simulink model "MR2_AndoidIPApplication"  (R2018b)
settings: Solver=VariableStepAuto  StartTime=0.0  StopTime=10.0  RelTol=1e-3
undefined symbols (not defined in the file): Backcamfinal, BLE_Send, LightIntensity, Line_Detection, LineDirection, Rec, SandDune, SDTV
libraries: androiduilib x8, androidaudiovideolib x2, visiontransforms x2, androidcommunicationlib x1, visionconversions x1, visionanalysis x1, visionstatistics x1, androidsensorlib x1, visiontextngfix x1
settings Model: Creator=Darshan  LastModifiedBy=Darshan

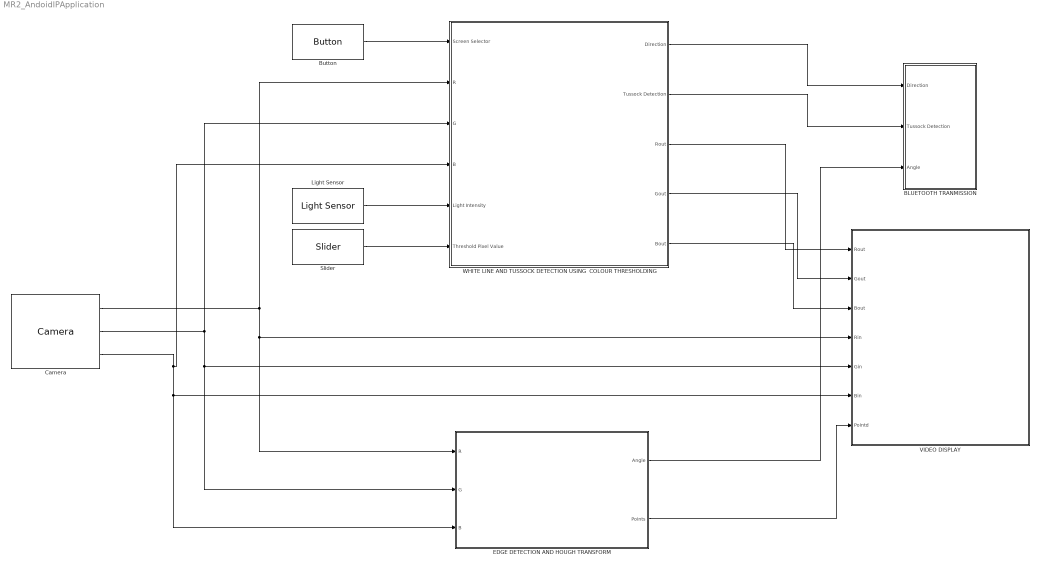
== system MR2_AndoidIPApplication ==
  BLUETOOTH TRANMISSION : Subsystem
  Button : androiduilib/Button  ButtonState=Not pressed  ButtonId=Backcamfinal/Button  State=off  SampleTime=0.1  BlockPlatform=Android
      settings: SourceProductName=Simulink Support Package for Android Devices  SourceProductBaseCode=ANDROID
  Camera : androidaudiovideolib/Camera  CameraLocation=Back  CameraResolutions=Back - 640x480  Width=640  Height=480  SampleTime=0.1  BlockPlatform=Android
      settings: SourceProductName=Simulink Support Package for Android Devices  SourceProductBaseCode=ANDROID
  "EDGE DETECTION AND HOUGH TRANSFORM " : Subsystem
  Light Sensor : androidsensorlib/Light Sensor  SampleTime=0.1  BlockPlatform=Android
      settings: SourceProductName=Simulink Support Package for Android Devices  SourceProductBaseCode=ANDROID
  Slider : androiduilib/Slider  Min=10000  Value=75000  Max=150000  Resolution=1  SliderId=Backcamfinal/Slider  SampleTime=0.1  BlockPlatform=Android
      settings: SourceProductName=Simulink Support Package for Android Devices  SourceProductBaseCode=ANDROID
  VIDEO DISPLAY : Subsystem
  WHITE LINE AND TUSSOCK DETECTION USING  COLOUR THRESHOLDING : Subsystem
  wires:
  "EDGE DETECTION AND HOUGH TRANSFORM "/2(Points) -> VIDEO DISPLAY/7(Pointd)
  WHITE LINE AND TUSSOCK DETECTION USING  COLOUR THRESHOLDING/5(Bout) -> VIDEO DISPLAY/3(Bout)
  WHITE LINE AND TUSSOCK DETECTION USING  COLOUR THRESHOLDING/3(Rout) -> VIDEO DISPLAY/1(Rout)
  WHITE LINE AND TUSSOCK DETECTION USING  COLOUR THRESHOLDING/2(Tussock Detection) -> BLUETOOTH TRANMISSION/2(Tussock Detection)
  WHITE LINE AND TUSSOCK DETECTION USING  COLOUR THRESHOLDING/1(Direction) -> BLUETOOTH TRANMISSION/1(Direction)
  Camera/3 -> "EDGE DETECTION AND HOUGH TRANSFORM "/3(B), VIDEO DISPLAY/6(Bin), WHITE LINE AND TUSSOCK DETECTION USING  COLOUR THRESHOLDING/4(B)
  Light Sensor/1 -> WHITE LINE AND TUSSOCK DETECTION USING  COLOUR THRESHOLDING/5(Light Intensity)
  Button/1 -> WHITE LINE AND TUSSOCK DETECTION USING  COLOUR THRESHOLDING/1(Screen Selector)
  Slider/1 -> WHITE LINE AND TUSSOCK DETECTION USING  COLOUR THRESHOLDING/6(Threshold Pixel Value)
  Camera/2 -> "EDGE DETECTION AND HOUGH TRANSFORM "/2(G), VIDEO DISPLAY/5(Gin), WHITE LINE AND TUSSOCK DETECTION USING  COLOUR THRESHOLDING/3(G)
  Camera/1 -> "EDGE DETECTION AND HOUGH TRANSFORM "/1(R), VIDEO DISPLAY/4(Rin), WHITE LINE AND TUSSOCK DETECTION USING  COLOUR THRESHOLDING/2(R)
  "EDGE DETECTION AND HOUGH TRANSFORM "/1("Angle ") -> BLUETOOTH TRANMISSION/3("Angle ")
  WHITE LINE AND TUSSOCK DETECTION USING  COLOUR THRESHOLDING/4(Gout) -> VIDEO DISPLAY/2(Gout)

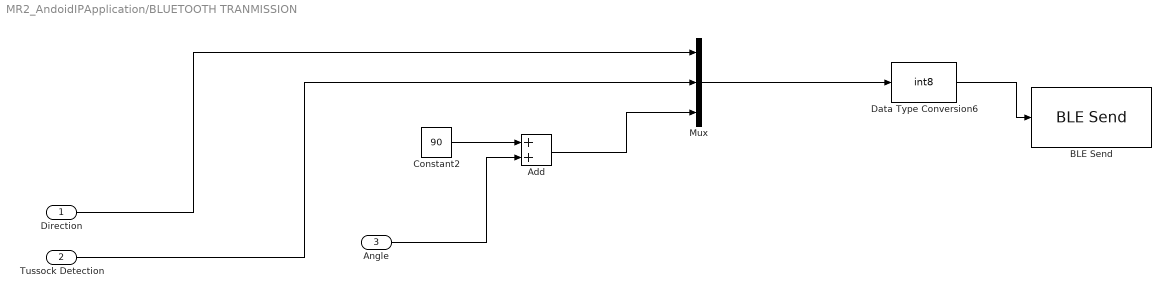
== system MR2_AndoidIPApplication/BLUETOOTH TRANMISSION ==
  Direction : Inport
  Tussock Detection : Inport  Port=2
  "Angle " : Inport  Port=3
  Add : Sum
  BLE Send : androidcommunicationlib/BLE Send  DeviceMode=Central (Client)  BluetoothAddress=00:15:85:14:9C:09  CharUUID=0000ffe1-0000-1000-8000-00805f9b34fb  ServiceUUID=0000ffe0-0000-1000-8000-00805f9b34fb  device=BT05  character=0000ffe0-0000-1000-8000-00805f9b34fb\0000ffe1-0000-1000-8000-00805f9b34fb  CustomService=off  ServiceName=Heart Rate  CharacteristicName="Heart Rate  Measurement"  CustomServiceUUID=<Enter Service UUID>  CustomCharUUID=<Enter Characteristic UUID>  charseruuid=00001800-0000-1000-8000-00805f9b34fb\00002a00-0000-1000-8000-00805f9b34fb  seruuid=00001810-0000-1000-8000-00805f9b34fb  chruuid=00002a37-0000-1000-8000-00805f9b34fb  PeripheralService=0000180d-0000-1000-8000-00805f9b34fb  PeripheralCharacteristic=00002a37-0000-1000-8000-00805f9b34fb  BLEId=Backcamfinal/BLE_Send  Devicename=BT05  IsCustomService=0  Size=-1
      settings: SourceProductName=Simulink Support Package for Android Devices  SourceProductBaseCode=ANDROID
  Constant2 : Constant  Value=90
  Data Type Conversion6 : DataTypeConversion  OutDataTypeStr=int8
  Mux : Mux  Inputs=3
  wires:
  Tussock Detection/1 -> Mux/2
  Constant2/1 -> Add/1
  Add/1 -> Mux/3
  Data Type Conversion6/1 -> BLE Send/1
  Direction/1 -> Mux/1
  Mux/1 -> Data Type Conversion6/1
  "Angle "/1 -> Add/2

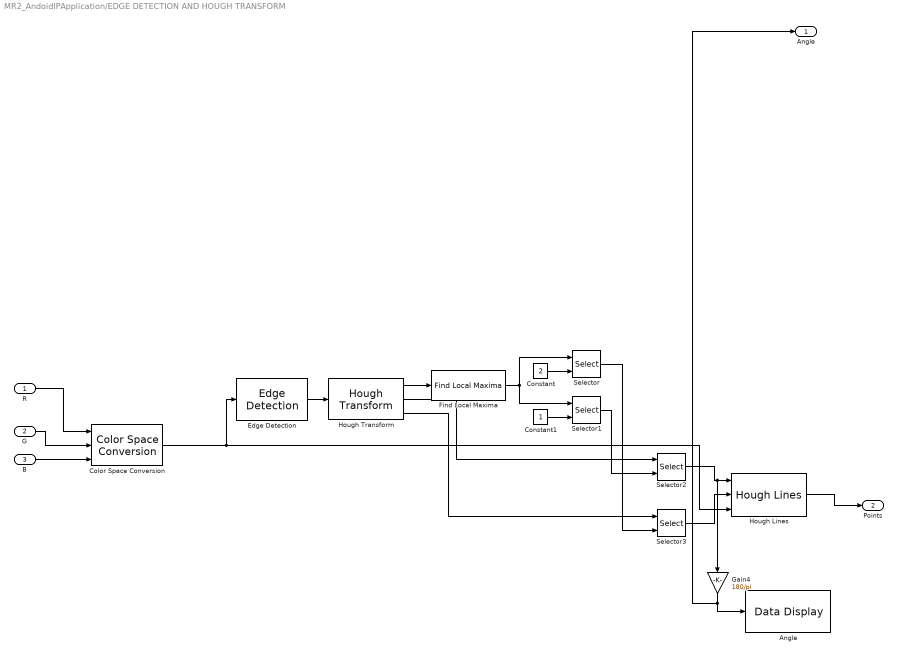
== system MR2_AndoidIPApplication/EDGE DETECTION AND HOUGH TRANSFORM  ==
  R : Inport
  G : Inport  Port=2
  B : Inport  Port=3
  Angle : androiduilib/Data Display  DataDisplayId=Backcamfinal/Angle  Format=Float  Precision=6  SimulateUsing=Code generation  blockPlatform=Android
      settings: SourceProductName=Simulink Support Package for Android Devices  SourceProductBaseCode=ANDROID
  Color Space Conversion : visionconversions/Color Space  Conversion  conversion=Obsolete  conversionActive=R'G'B' to intensity  wp_str=D65  rec=Rec. 601 (SDTV)  sys=1125/60/2:1  imagePorts=Separate color signals
      settings: SourceProductName=Computer Vision System Toolbox
  Constant : Constant  Value=2
  Constant1 : Constant
  Edge Detection : visionanalysis/Edge Detection  method=Sobel  outputType=Binary image  userDefinedThreshold=off  thresholdSource=Input port  threshold=20  thresholdTuning=10  edgeThinning=off  threshold_canny=[0.25 0.60]  autoPercent=70  sigma=1  roundingMode=Floor  overflowMode=off  prodOutputMode=Binary point scaling  prodOutputWordLength=32  prodOutputFracLength=8  prodOutputSlope=2^-8  accumSlope=2^-8  outputSlope=2^-4
      settings: SourceProductName=Computer Vision System Toolbox  SourceProductBaseCode=VP
  Find Local Maxima : visionstatistics/Find Local Maxima  num_peaks=1  nhood_size=[5 7]  src_thresh=Obsolete9b  src_thresh_inuse=Specify via dialog  threshold=10  inputIsHough=on  dt_peak=uint32  isOutVarDim=on  dt_count=uint32
      settings: SourceProductName=Computer Vision System Toolbox  SourceProductBaseCode=VP
  Gain4 : Gain  Gain=180/pi
  Hough Lines : visiontransforms/Hough Lines  sineCompMethod=Trigonometric function  thetaRes=pi/180  firstCoeffMode=Specify word length  firstCoeffWordLength=16  firstCoeffFracLength=15  prodOutputMode=Binary point scaling  prodOutputWordLength=32  prodOutputFracLength=16  roundingMode=Nearest  overflowMode=on
      settings: SourceProductName=Computer Vision System Toolbox  SourceProductBaseCode=VP
  Hough Transform : visiontransforms/Hough Transform  theta_res=pi/360  rho_res=1  out_theta_rho=on  outdtmode=double  roundingMode=Nearest  overflowMode=on  firstCoeffMode=Binary point scaling  firstCoeffWordLength=16  firstCoeffFracLength=14  firstCoeffSlope=2^-14  secondCoeffMode=Binary point scaling  secondCoeffWordLength=32  secondCoeffFracLength=16  secondCoeffSlope=2^-16  prodOutputMode=Binary point scaling  prodOutputWordLength=32  prodOutputFracLength=20  prodOutputSlope=2^-20  accumMode=Binary point scaling  accumWordLength=32  accumFracLength=20  accumSlope=2^-20  outputMode=Binary point scaling  outputWordLength=16  outputFracLength=0  outputSlope=2^0  memoryMode=Binary point scaling  memoryWordLength=32  memoryFracLength=16  memorySlope=2^-16
      settings: SourceProductName=Computer Vision System Toolbox  SourceProductBaseCode=VP
  Selector : Selector  InputPortWidth=2  IndexOptions=Index vector (port)  Indices=1  OutputSizes=1
  Selector1 : Selector  InputPortWidth=2  IndexOptions=Index vector (port)  Indices=0  OutputSizes=1
  Selector2 : Selector  NumberOfDimensions=2  InputPortWidth=3  IndexOptions=Select all,Index vector (port)  Indices=[1 3],1  OutputSizes=1,1
  Selector3 : Selector  NumberOfDimensions=2  InputPortWidth=3  IndexOptions=Select all,Index vector (port)  Indices=[1 3],1  OutputSizes=1,1
  "Angle " : Outport
  Points : Outport  Port=2
  wires:
  Edge Detection/1 -> Hough Transform/1
  Constant/1 -> Selector/2
  Color Space Conversion/1 -> Hough Lines/3, Edge Detection/1
  Hough Transform/2 -> Selector2/1
  Selector/1 -> Selector3/2
  Selector1/1 -> Selector2/2
  Hough Transform/3 -> Selector3/1
  Constant1/1 -> Selector1/2
  Find Local Maxima/1 -> Selector1/1, Selector/1
  Hough Transform/1 -> Find Local Maxima/1
  Selector2/1 -> Gain4/1, Hough Lines/1
  Gain4/1 -> Angle/1, "Angle "/1
  Selector3/1 -> Hough Lines/2
  R/1 -> Color Space Conversion/1
  G/1 -> Color Space Conversion/2
  B/1 -> Color Space Conversion/3
  Hough Lines/1 -> Points/1

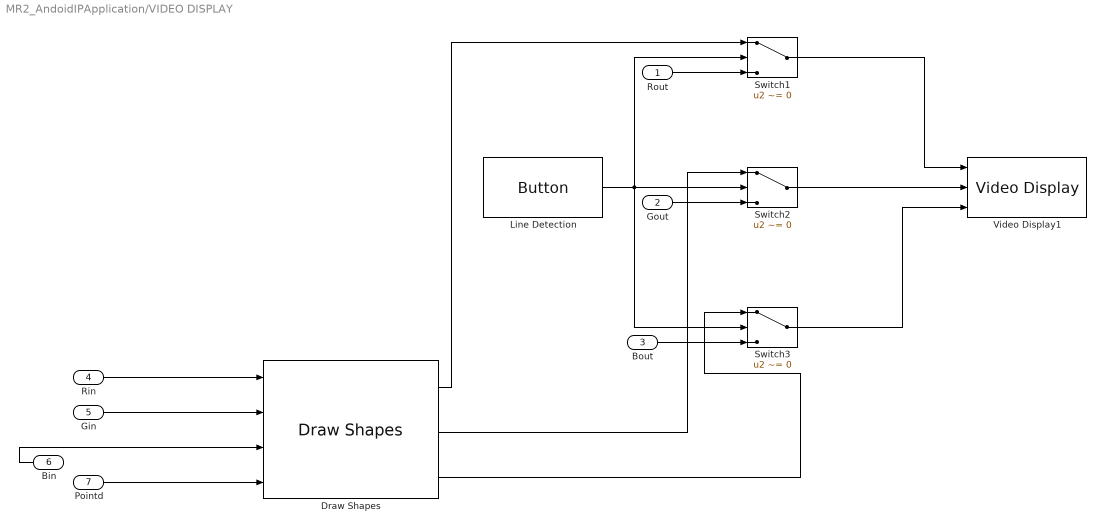
== system MR2_AndoidIPApplication/VIDEO DISPLAY ==
  Rout : Inport
  Gout : Inport  Port=2
  Bout : Inport  Port=3
  Rin : Inport  Port=4
  Gin : Inport  Port=5
  Bin : Inport  Port=6
  Pointd : Inport  Port=7
  Draw Shapes : visiontextngfix/Draw Shapes  shape=Lines  fill=off  lineWidth=5  fillClrSource=Specify via dialog  display=User-specified value  intensity=200  color=[0 255 0]  opacity=0.6  viewport=Entire image  antialiasing=off  inType=Obsolete  imagePorts=Separate color signals  prodOutputMode=Binary point scaling  prodOutputWordLength=32  prodOutputFracLength=14  memoryMode=Specify word length  memoryWordLength=16  memoryFracLength=14  roundingMode=Floor  overflowMode=off
      settings: SourceProductName=Computer Vision System Toolbox
  Line Detection : androiduilib/Button  ButtonState=Not pressed  ButtonId=Backcamfinal/Line_Detection  State=off  SampleTime=0.1  BlockPlatform=Android
      settings: SourceProductName=Simulink Support Package for Android Devices  SourceProductBaseCode=ANDROID
  Switch1 : Switch  Criteria=u2 ~= 0
  Switch2 : Switch  Criteria=u2 ~= 0
  Switch3 : Switch  Criteria=u2 ~= 0
  Video Display1 : androidaudiovideolib/Video Display  BlockPlatform=Android
      settings: SourceProductName=Simulink Support Package for Android Devices  SourceProductBaseCode=ANDROID
  wires:
  Switch1/1 -> Video Display1/1
  Switch3/1 -> Video Display1/3
  Gin/1 -> Draw Shapes/2
  Switch2/1 -> Video Display1/2
  Line Detection/1 -> Switch1/2, Switch2/2, Switch3/2
  Rin/1 -> Draw Shapes/1
  Draw Shapes/2 -> Switch2/1
  Draw Shapes/1 -> Switch1/1
  Draw Shapes/3 -> Switch3/1
  Pointd/1 -> Draw Shapes/4
  Rout/1 -> Switch1/3
  Bout/1 -> Switch3/3
  Gout/1 -> Switch2/3
  Bin/1 -> Draw Shapes/3

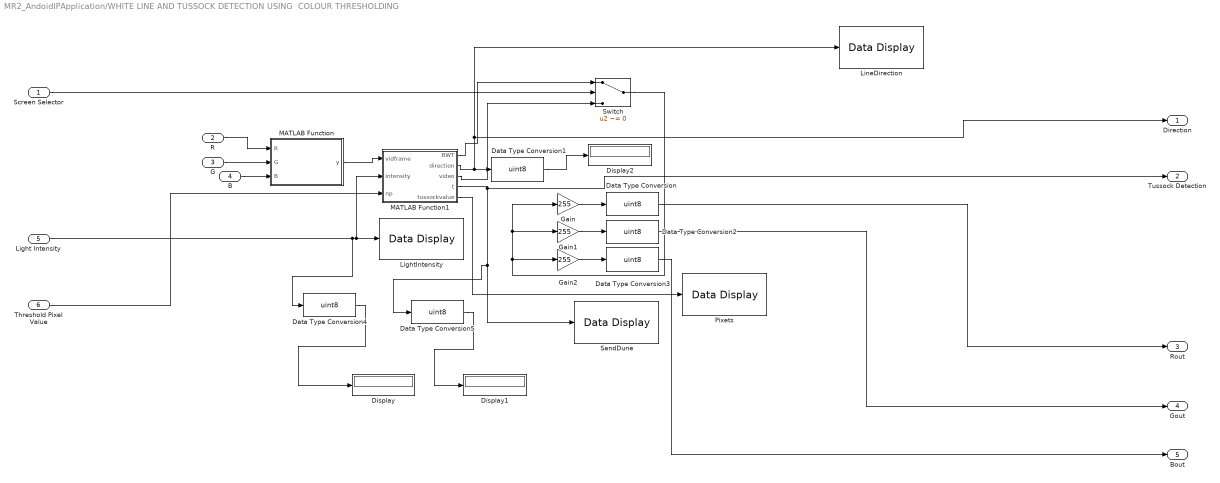
== system MR2_AndoidIPApplication/WHITE LINE AND TUSSOCK DETECTION USING  COLOUR THRESHOLDING ==
  Screen Selector : Inport
  R : Inport  Port=2
  G : Inport  Port=3
  B : Inport  Port=4
  Light Intensity : Inport  Port=5
  Threshold Pixel Value : Inport  Port=6
  Data Type Conversion{,1..5} (6 alike) : DataTypeConversion  OutDataTypeStr=uint8
  Display : Display
  Display1 : Display
  Display2 : Display
  Gain : Gain  Gain=255
  Gain1 : Gain  Gain=255
  Gain2 : Gain  Gain=255
  LightIntensity : androiduilib/Data Display  DataDisplayId=Backcamfinal/LightIntensity  Format=Float  Precision=6  SimulateUsing=Code generation  blockPlatform=Android
      settings: SourceProductName=Simulink Support Package for Android Devices  SourceProductBaseCode=ANDROID
  LineDirection : androiduilib/Data Display  DataDisplayId=Backcamfinal/LineDirection  Format=Float  Precision=6  SimulateUsing=Code generation  blockPlatform=Android
      settings: SourceProductName=Simulink Support Package for Android Devices  SourceProductBaseCode=ANDROID
  MATLAB Function : MATLAB Function  TreatAsAtomicUnit=on
  MATLAB Function1 : MATLAB Function  TreatAsAtomicUnit=on
  Pixets : androiduilib/Data Display  DataDisplayId=Backcamfinal/Pixets  Format=Float  Precision=6  SimulateUsing=Code generation  blockPlatform=Android
      settings: SourceProductName=Simulink Support Package for Android Devices  SourceProductBaseCode=ANDROID
  SandDune : androiduilib/Data Display  DataDisplayId=Backcamfinal/SandDune  Format=Float  Precision=6  SimulateUsing=Code generation  blockPlatform=Android
      settings: SourceProductName=Simulink Support Package for Android Devices  SourceProductBaseCode=ANDROID
  Switch : Switch  Criteria=u2 ~= 0
  Direction : Outport
  Tussock Detection : Outport  Port=2
  Rout : Outport  Port=3
  Gout : Outport  Port=4
  Bout : Outport  Port=5
  wires:
  Switch/1 -> Gain/1, Gain1/1, Gain2/1
  Screen Selector/1 -> Switch/2
  Light Intensity/1 -> Data Type Conversion4/1, LightIntensity/1, MATLAB Function1/2(intensity)
  Gain1/1 -> Data Type Conversion2/1
  MATLAB Function1/1(BWT) -> Switch/1
  MATLAB Function/1(y) -> MATLAB Function1/1(vidframe)
  MATLAB Function1/4(t) -> Tussock Detection/1, Data Type Conversion5/1, SandDune/1
  Data Type Conversion/1 -> Rout/1
  MATLAB Function1/2(direction) -> Direction/1, LineDirection/1, Data Type Conversion1/1
  MATLAB Function1/5(tussockvalue) -> Pixets/1
  Gain/1 -> Data Type Conversion/1
  Data Type Conversion3/1 -> Bout/1
  Data Type Conversion2/1 -> Gout/1
  Data Type Conversion4/1 -> Display/1
  MATLAB Function1/3(video) -> Switch/3
  Data Type Conversion5/1 -> Display1/1
  Gain2/1 -> Data Type Conversion3/1
  Data Type Conversion1/1 -> Display2/1
  R/1 -> MATLAB Function/1(R)
  Threshold Pixel Value/1 -> MATLAB Function1/3(np)
  G/1 -> MATLAB Function/2(G)
  B/1 -> MATLAB Function/3(B)

== matlab function MR2_AndoidIPApplication/WHITE LINE AND TUSSOCK DETECTION USING  COLOUR THRESHOLDING/MATLAB Function1 ==
  data: BWT output; vidframe input; direction output; intensity input; video output; t output; np input; tussockvalue output
function [BWT,direction,video,t,tussockvalue] = fcn(vidframe,intensity,np)   
I=rgb2hsv(vidframe);
% Define thresholds for channel 1 based on histogram settings
channel1Min = 0.084;
channel1Max = 0.226;

% Define thresholds for channel 2 based on histogram settings
channel2Min = 0.10;
channel2Max = 0.401;

% Define thresholds for channel 3 based on histogram settings
channel3Min = 0.608;
channel3Max = 0.886;

% Create mask based on chosen histogram thresholds
sliderBW = (I(:,:,1) >= channel1Min ) & (I(:,:,1) <= channel1Max) & ...
    (I(:,:,2) >= channel2Min ) & (I(:,:,2) <= channel2Max) & ...
    (I(:,:,3) >= channel3Min ) & (I(:,:,3) <= channel3Max);
BWT = sliderBW;
A=0;
% BW1 = bwareaopen(sliderBW,550);
for i=1:51200*6
   if BWT(i)==1
    A=A+1;
   end
end

if A>np 
    z=11;
else
    z=00;
end


channel1Min = 0.172;
channel1Max = 0.697;

% Define thresholds for channel 2 based on histogram settings
channel2Min = 0.099;
channel2Max = 0.578;

% Define thresholds for channel 3 based on histogram settings
channel3Min = 0.611;
channel3Max = 1.000;

% Create mask based on chosen histogram thresholds
BW1 = (I(:,:,1) >= channel1Min ) & (I(:,:,1) <= channel1Max) & ...
    (I(:,:,2) >= channel2Min ) & (I(:,:,2) <= channel2Max) & ...
    (I(:,:,3) >= channel3Min ) & (I(:,:,3) <= channel3Max);
%BWA = bwareaopen(BW,200);
%Edge = edge(BW,'canny');
%   BW1 = imfill(BW,'holes');
  %%step(vidPlayer,BW);
  %%step(vidPlayer,Edge);
  %count(640)=0;
   sum1=0;
   sum2=0;
   sum3=0;
   sum4=0;
   sum5=0;
% count(1)=0;
%%int sum[3];
%%int k=0;  a
 for i =1:51200 
     if BW1(i)==1
         sum1=sum1+1;
  end
end
for i=51201:(51200*2)
    if BW1(i)==1
       sum2=sum2+1;
    end
end
for i=((51200*2)+1):(51200*4)
    if BW1(i)==1
        sum3=sum3+1;
    end
end

for i=((51200*4)+1):(51200*5)
    if BW1(i)==1
        sum4=sum4+1;
    end
end


for i=((51200*5)+1):(51200*6)
    if BW1(i)==1
        sum5=sum5+1;
    end
end

X = [sum1 sum2 sum3 sum4 sum5]; 
Maximum=max(X);
[a,b] = max(X);
%u=b;
%disp(b)
tussockvalue=A;
t=z;
video = BW1;
direction = b;

== matlab function MR2_AndoidIPApplication/WHITE LINE AND TUSSOCK DETECTION USING  COLOUR THRESHOLDING/MATLAB Function ==
  data: R input; y output; G input; B input
function y = fcn(R,G,B)
I = cat(3,R,G,B);

y = I;
